simulink model "GFM_29bus"  (R2021a)
settings: Solver=ode1  StartTime=0.0  StopTime=4.5  FixedStep=Time_Step  RelTol=1e-3  EnableMultiTasking=on
PreLoadFcn:
  | Init_29bus;
InitFcn:
  | Init_29bus;
undefined symbols (not defined in the file): D1, D11, Delta, Time_Step, VSC01_Delta_P_Time_Step, VSC01_Delta_P_Value
libraries: spsSeriesRLCBranchLib x41, spsLoadFlowBusLib x28, spsDistributedParametersLineLib x19, spsThreePhaseSeriesRLCLoadLib x15, spsThreePhaseTransformerTwoWindingsLib x12, spsThreePhaseVIMeasurementLib x11, spsThreePhaseParallelRLCLoadLib x10, spsSynchronousMachinepuStandardLib x6, spsExcitationSystemLib x6, spsHydraulicTurbineandGovernorLib x6, spsGenericPowerSystemStabilizerLib x6, spsMultiBandPowerSystemStabilizerLib x6
(part 5 of 6)

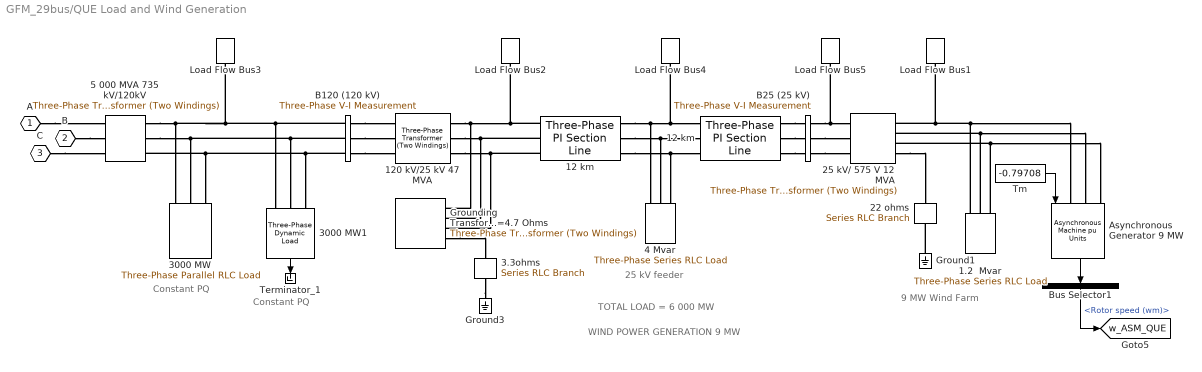
== system GFM_29bus/QUE Load and Wind Generation ==
  note: 9 MW Wind Farm
  note: 25 kV feeder
  note: Constant PQ
  note: Constant PQ
  note: WIND POWER GENERATION 9 MW
  note: TOTAL LOAD = 6 000 MW
  1.2  Mvar : spsThreePhaseSeriesRLCLoadLib/Three-Phase Series RLC Load  LConnTagsString=A|B|C  Configuration=Delta  NominalVoltage=575  Vabc=[1e3 1e3 1e3]  Vabcp=[1e3 1e3 1e3]  NominalFrequency=60  UnbalancedPower=off  ActivePower=1.2e6/50  InductivePower=0  CapacitivePower=1.2e6  Pabc=[10e3 9e3 11e3]  QLabc=[100 90 110]  QCabc=[100 90 110]  Pabcp=[10e3 9e3 11e3]  QLabcp=[100 90 110]  QCabcp=[100 90 110]  Measurements=None  LoadType=constant Z
  12 km : spsThreePhasePISectionLineLib/Three-Phase PI Section Line  LConnTagsString=a|b|c  RConnTagsString=A|B|C  Length=12  Frequency=60  Resistances=[0.1153 0.413]  Inductances=[1.05e-3 3.32e-3]  Capacitances=[11.33e-009 5.01e-009]
  "12 km " : spsThreePhasePISectionLineLib/Three-Phase PI Section Line  LConnTagsString=a|b|c  RConnTagsString=A|B|C  Length=12  Frequency=60  Resistances=[0.1153 0.413]  Inductances=[1.05e-3 3.32e-3]  Capacitances=[11.33e-009 5.01e-009]
  120 kV/25 kV 47 MVA : spsThreePhaseTransformerTwoWindingsLib/Three-Phase Transformer (Two Windings)  Winding1Connection=Yg  Winding2Connection=Delta (D1)  CoreType=Three single-phase transformers  SetSaturation=off  Hysteresis=off  DataFile='basic_model'  SetInitialFlux=off  Measurements=None  UNITS=pu  NominalPower=[47e6 60 ]  Winding1="[ 120e3  0.08/30   0.08 ]"  Winding2="[ 25e3  0.08/30  0.08]"  Rm=500  Lm=500  L0=0.5  Saturation="[ 0,0  ;  0.005,1.2  ;  1.0,1.4 ]"  InitialFluxes=[ 0.8 , -0.8 , 0.7 ]  BreakLoop=off  DiscreteSolver=Trapezoidal iterative  DataType=off  TransfoNumber=0
  "22 ohms " : spsSeriesRLCBranchLib/Series RLC Branch  LConnTagsString=__new0  RConnTagsString=__new0  BranchType=R  Resistance=22  Inductance=1.0  SetiL0=off  InitialCurrent=0  Capacitance=1.0  Setx0=off  InitialVoltage=0  Measurements=None
  25 kV/ 575 V 12 MVA : spsThreePhaseTransformerTwoWindingsLib/Three-Phase Transformer (Two Windings)  Winding1Connection=Yg  Winding2Connection=Yn  CoreType=Three single-phase transformers  SetSaturation=off  Hysteresis=off  DataFile='hysteresis'  SetInitialFlux=off  Measurements=None  UNITS=pu  NominalPower="[12e6  60]"  Winding1=[25e3 , 0.025/30 , 0.025]  Winding2=[ 575, 0.025/30 , 0.025]  Rm=500  Lm=inf  L0=0.5  Saturation=[ 0,0 ; 0.0024,1.2 ; 1.0,1.52 ]  InitialFluxes=[ 0.8 , -0.8 , 0.7 ]  BreakLoop=off  DiscreteSolver=Trapezoidal iterative  DataType=off  TransfoNumber=0
  "3.3ohms " : spsSeriesRLCBranchLib/Series RLC Branch  LConnTagsString=__new0  RConnTagsString=__new0  BranchType=R  Resistance=3.3  Inductance=1.0  SetiL0=off  InitialCurrent=0  Capacitance=1.0  Setx0=off  InitialVoltage=0  Measurements=None
  3000 MW : spsThreePhaseParallelRLCLoadLib/Three-Phase Parallel RLC Load  LConnTagsString=A|B|C  Configuration=Y (grounded)  NominalVoltage=(120000)*1.0062  Vabc=[1e3 1e3 1e3]  Vabcp=[1e3 1e3 1e3]  NominalFrequency=60  UnbalancedPower=off  ActivePower=3000000000  InductivePower=0  CapacitivePower=0  Pabc=[10e3 9e3 11e3]  QLabc=[100 90 110]  QCabc=[100 90 110]  Pabcp=[10e3 9e3 11e3]  QLabcp=[100 90 110]  QCabcp=[100 90 110]  Measurements=None  LoadType=constant PQ
  3000 MW1 : spsThreePhaseDynamicLoadLib/Three-Phase Dynamic Load  NominalVoltage=[ 120e3 60 ]  ActiveReactivePowers=[3e+09 0]  PositiveSequence=[1.0062 -46.9013]  ExternalControl=off  NpNq=[1.3 2]  TimeConstants="[0  0  0  0]"  MinimumVoltage=0.7  Tfilter=1e-4  LoadFlowParameters=[4,0,0,0,0]
      settings: SourceProductBaseCode=PS
  4 Mvar : spsThreePhaseSeriesRLCLoadLib/Three-Phase Series RLC Load  LConnTagsString=A|B|C  Configuration=Delta  NominalVoltage=25e3  Vabc=[1e3 1e3 1e3]  Vabcp=[1e3 1e3 1e3]  NominalFrequency=60  UnbalancedPower=off  ActivePower=0  InductivePower=0  CapacitivePower=4e6  Pabc=[10e3 9e3 11e3]  QLabc=[100 90 110]  QCabc=[100 90 110]  Pabcp=[10e3 9e3 11e3]  QLabcp=[100 90 110]  QCabcp=[100 90 110]  Measurements=None  LoadType=constant Z
  5 000 MVA 735 kV/120kV : spsThreePhaseTransformerTwoWindingsLib/Three-Phase Transformer (Two Windings)  Winding1Connection=Yg  Winding2Connection=Delta (D1)  CoreType=Three single-phase transformers  SetSaturation=off  Hysteresis=off  DataFile='basic_model'  SetInitialFlux=off  Measurements=None  UNITS=pu  NominalPower=[ 5000e6 60 ]  Winding1="[ 735e3 0.002  0.12]"  Winding2=[120e3 0.002 0]  Rm=500  Lm=500  L0=0.5  Saturation="[ 0,0  ;  0.005,1.2  ;  1.0,1.4 ]"  InitialFluxes=[ 0.8 , -0.8 , 0.7 ]  BreakLoop=off  DiscreteSolver=Trapezoidal iterative  DataType=off  TransfoNumber=0
  Asynchronous Generator 9 MW : spsAsynchronousMachinepuUnitsLib/Asynchronous Machine pu Units  RotorType=Squirrel-cage  PresetModel=No  MechanicalLoad=Torque Tm  ShowDetailedParameters=on  ReferenceFrame=Rotor  Units=pu  MeasurementBus=off  NominalParameters=[6*1.5e6/0.9 575 60]  VoltageRatio=1  Stator=[ 0.004843 0.1248]  Rotor=[ 0.004377 0.1791]  Cage1=[0.01909 0.0397]  Cage2=[0.01909 0.0397]  Lm=6.77  Mechanical="[5.04  0  3]"  PolePairs=3  InitialConditions=[-0.00366846 0 0.851241 0.851241 0.851241 136.952 16.9521 256.952]  SimulateSaturation=off  Saturation=[ 0 0 ; 0 0 ]  LoadFlowParameters=0  TsPowergui=0  TsBlock=-1  IterativeModel=Trapezoidal non iterative  IterativeDiscreteModel=Trapezoidal non iterative  Pmec=-8000000
      settings: SourceProductBaseCode=PS
  B120 (120 kV) : spsThreePhaseVIMeasurementLib/Three-Phase V-I Measurement  VoltageMeasurement=no  SetLabelV=on  LabelV=Vabc_B120  Vpu=on  VpuLL=off  CurrentMeasurement=no  SetLabelI=on  LabelI=Iabc_B120  Ipu=off  Pbase=100e6  Vbase=120e3  OutputType=Complex  PhasorSimulation=off  PSBequivalent=0
  B25 (25 kV) : spsThreePhaseVIMeasurementLib/Three-Phase V-I Measurement  VoltageMeasurement=no  SetLabelV=on  LabelV=Vabc_B25  Vpu=on  VpuLL=off  CurrentMeasurement=no  SetLabelI=on  LabelI=Iabc_B25  Ipu=on  Pbase=10e6  Vbase=25e3  OutputType=Complex  PhasorSimulation=off  PSBequivalent=0
  Bus Selector1 : BusSelector  OutputSignals=Mechanical.Rotor speed (wm)
  Ground1 : spsGroundLib/Ground  LConnTagsString=a
  Ground3 : spsGroundLib/Ground  LConnTagsString=a
  Grounding Transformer X0=4.7 Ohms : spsThreePhaseTransformerTwoWindingsLib/Three-Phase Transformer (Two Windings)  Winding1Connection=Yn  Winding2Connection=Delta (D11)  CoreType=Three single-phase transformers  SetSaturation=off  Hysteresis=off  DataFile='basic_model'  SetInitialFlux=off  Measurements=None  UNITS=pu  NominalPower=[100e6 60]  Winding1="[ 25e3  4.7/(25e3^2/100e6)/30    4.7/(25e3^2/100e6)]"  Winding2="[ 25e3  1e-6  0]"  Rm=500  Lm=500  L0=0.5  Saturation="[ 0,0  ;  0.005,1.2  ;  1.0,1.4 ]"  InitialFluxes=[ 0.8 , -0.8 , 0.7 ]  BreakLoop=off  DiscreteSolver=Trapezoidal iterative  DataType=off  TransfoNumber=0
  Load Flow Bus1 : spsLoadFlowBusLib/Load Flow Bus  LConnTagsString=a  Phases=single  Connectors=on one side  ID=QUE_575  Vbase=575  Vref=1  Vangle=0  VLF=1.021  VLFb=1  VLFc=1  angleLF=-67.07  angleLFb=0  angleLFc=0
      settings: AttributesFormatString=%<ID>\n%<Vbase>V\n%<VLF>pu\n%<angleLF>deg.  SourceProductBaseCode=PS
  Load Flow Bus2 : spsLoadFlowBusLib/Load Flow Bus  LConnTagsString=a  Phases=single  Connectors=on one side  ID=QUE_25_1  Vbase=25e3  Vref=1  Vangle=0  VLF=1.009  VLFb=1  VLFc=1  angleLF=-75.49  angleLFb=0  angleLFc=0
      settings: AttributesFormatString=%<ID>\n%<Vbase>V\n%<VLF>pu\n%<angleLF>deg.  SourceProductBaseCode=PS
  Load Flow Bus3 : spsLoadFlowBusLib/Load Flow Bus  LConnTagsString=a  Phases=single  Connectors=on one side  ID=QUE1  Vbase=120e3  Vref=1  Vangle=0  VLF=1.006  VLFb=1  VLFc=1  angleLF=-46.9  angleLFb=0  angleLFc=0
      settings: AttributesFormatString=%<ID>\n%<Vbase>V\n%<VLF>pu\n%<angleLF>deg.  SourceProductBaseCode=PS
  Load Flow Bus4 : spsLoadFlowBusLib/Load Flow Bus  LConnTagsString=a  Phases=single  Connectors=on one side  ID=QUE_25_2  Vbase=25e3  Vref=1  Vangle=0  VLF=1.033  VLFb=1  VLFc=1  angleLF=-72.41  angleLFb=0  angleLFc=0
      settings: AttributesFormatString=%<ID>\n%<Vbase>V\n%<VLF>pu\n%<angleLF>deg.  SourceProductBaseCode=PS
  Load Flow Bus5 : spsLoadFlowBusLib/Load Flow Bus  LConnTagsString=a  Phases=single  Connectors=on one side  ID=QUE_25_3  Vbase=25e3  Vref=1  Vangle=0  VLF=1.029  VLFb=1  VLFc=1  angleLF=-68.88  angleLFb=0  angleLFc=0
      settings: AttributesFormatString=%<ID>\n%<Vbase>V\n%<VLF>pu\n%<angleLF>deg.  SourceProductBaseCode=PS
  Terminator_1 : Terminator
  Tm : Constant  Value=-0.79708
  A : PMIOPort  Side=Left
  B : PMIOPort  Port=2  Side=Left
  C : PMIOPort  Port=3  Side=Left
  tag scope: w_ASM_QUE=global
  wires:
  Tm/1 -> Asynchronous Generator 9 MW/1
  Asynchronous Generator 9 MW/1 -> Bus Selector1/1
  Bus Selector1/1 -> [w_ASM_QUE]  "<Rotor speed (wm)>"
  3000 MW1/1 -> Terminator_1/1
  connections:
  B120 (120 kV)/RConn3 -- 120 kV/25 kV 47 MVA/LConn3
  B120 (120 kV)/RConn2 -- 120 kV/25 kV 47 MVA/LConn2
  B120 (120 kV)/RConn1 -- 120 kV/25 kV 47 MVA/LConn1
  A/RConn1 -- 5 000 MVA 735 kV/120kV/LConn1
  B/RConn1 -- 5 000 MVA 735 kV/120kV/LConn2
  C/RConn1 -- 5 000 MVA 735 kV/120kV/LConn3
  Load Flow Bus3/LConn1 -- B120 (120 kV)/LConn1 -- 3000 MW1/LConn1 -- 5 000 MVA 735 kV/120kV/RConn1 -- 3000 MW/LConn1
  B120 (120 kV)/LConn2 -- 5 000 MVA 735 kV/120kV/RConn2 -- 3000 MW/LConn2 -- 3000 MW1/LConn2
  B120 (120 kV)/LConn3 -- 5 000 MVA 735 kV/120kV/RConn3 -- 3000 MW/LConn3 -- 3000 MW1/LConn3
  12 km/LConn2 -- 120 kV/25 kV 47 MVA/RConn2 -- Grounding Transformer X0=4.7 Ohms/LConn2
  12 km/LConn3 -- 120 kV/25 kV 47 MVA/RConn3 -- Grounding Transformer X0=4.7 Ohms/LConn3
  Load Flow Bus2/LConn1 -- 12 km/LConn1 -- Grounding Transformer X0=4.7 Ohms/LConn1 -- 120 kV/25 kV 47 MVA/RConn1
  "3.3ohms "/RConn1 -- Ground3/LConn1
  Grounding Transformer X0=4.7 Ohms/LConn4 -- "3.3ohms "/LConn1
  25 kV/ 575 V 12 MVA/RConn4 -- "22 ohms "/LConn1
  Ground1/LConn1 -- "22 ohms "/RConn1
  Load Flow Bus1/LConn1 -- 1.2  Mvar/LConn1 -- Asynchronous Generator 9 MW/LConn1 -- 25 kV/ 575 V 12 MVA/RConn1
  1.2  Mvar/LConn2 -- 25 kV/ 575 V 12 MVA/RConn2 -- Asynchronous Generator 9 MW/LConn2
  1.2  Mvar/LConn3 -- 25 kV/ 575 V 12 MVA/RConn3 -- Asynchronous Generator 9 MW/LConn3
  B25 (25 kV)/RConn1 -- 25 kV/ 575 V 12 MVA/LConn1 -- Load Flow Bus5/LConn1
  B25 (25 kV)/RConn2 -- 25 kV/ 575 V 12 MVA/LConn2
  B25 (25 kV)/RConn3 -- 25 kV/ 575 V 12 MVA/LConn3
  "12 km "/RConn1 -- B25 (25 kV)/LConn1
  "12 km "/RConn2 -- B25 (25 kV)/LConn2
  "12 km "/RConn3 -- B25 (25 kV)/LConn3
  12 km/RConn1 -- "12 km "/LConn1 -- Load Flow Bus4/LConn1 -- 4 Mvar/LConn1
  12 km/RConn2 -- "12 km "/LConn2 -- 4 Mvar/LConn2
  12 km/RConn3 -- "12 km "/LConn3 -- 4 Mvar/LConn3

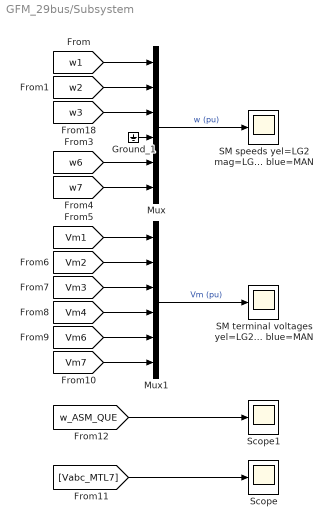
== system GFM_29bus/Subsystem ==
  Ground_1 : Ground
  Mux : Mux  Inputs=6
  Mux1 : Mux  Inputs=6
  "SM speeds yel=LG2 mag=LG3 cyan=LG4 red=MTL green=CHU blue=MAN " : Scope
  SM terminal voltages yel=LG2 mag=LG3 cyan=LG4 red=MTL green=CHU blue=MAN : Scope
  Scope : Scope
  Scope1 : Scope
  wires:
  [Vabc_MTL7] -> Scope/1
  [w_ASM_QUE] -> Scope1/1
  Mux/1 -> "SM speeds yel=LG2 mag=LG3 cyan=LG4 red=MTL green=CHU blue=MAN "/1  "w (pu)"
  [w1] -> Mux/1
  [w2] -> Mux/2
  [w7] -> Mux/6
  [w6] -> Mux/5
  [w3] -> Mux/3
  Mux1/1 -> SM terminal voltages yel=LG2 mag=LG3 cyan=LG4 red=MTL green=CHU blue=MAN/1  "Vm (pu)"
  [Vm1] -> Mux1/1
  [Vm2] -> Mux1/2
  [Vm7] -> Mux1/6
  [Vm6] -> Mux1/5
  [Vm4] -> Mux1/4
  [Vm3] -> Mux1/3
  Ground_1/1 -> Mux/4

== system GFM_29bus/Subsystem1 ==
  In1 : Inport
  Constant : Constant
  Sum : Sum  Inputs=|++  SaturateOnIntegerOverflow=on
  tag scope: PSS_select=global
  wires:
  In1/1 -> Sum/1
  Sum/1 -> [PSS_select]
  Constant/1 -> Sum/2

== system GFM_29bus/Subsystem2 ==

== system GFM_29bus/North-West Network/Cs  CHMN  ==
  note: B
  Ca : spsSeriesRLCBranchLib/Series RLC Branch  LConnTagsString=__new0  RConnTagsString=__new0  BranchType=C  Resistance=1.0  Inductance=1.0  SetiL0=off  InitialCurrent=0  Capacitance=Cs  Setx0=off  InitialVoltage=0  Measurements=None
  Cb : spsSeriesRLCBranchLib/Series RLC Branch  LConnTagsString=__new0  RConnTagsString=__new0  BranchType=C  Resistance=1.0  Inductance=1.0  SetiL0=off  InitialCurrent=0  Capacitance=Cs  Setx0=off  InitialVoltage=0  Measurements=None
  Cc : spsSeriesRLCBranchLib/Series RLC Branch  LConnTagsString=__new0  RConnTagsString=__new0  BranchType=C  Resistance=1.0  Inductance=1.0  SetiL0=off  InitialCurrent=0  Capacitance=Cs  Setx0=off  InitialVoltage=0  Measurements=None
  A : PMIOPort  Side=Left
  B : PMIOPort  Port=2  Side=Left
  C : PMIOPort  Port=3  Side=Left
  "A " : PMIOPort  Port=4  Side=Right
  "B " : PMIOPort  Port=5  Side=Right
  "C " : PMIOPort  Port=6  Side=Right
  connections:
  Cc/RConn1 -- "C "/RConn1
  C/RConn1 -- Cc/LConn1
  Cb/RConn1 -- "B "/RConn1
  B/RConn1 -- Cb/LConn1
  Ca/RConn1 -- "A "/RConn1
  A/RConn1 -- Ca/LConn1

== system GFM_29bus/North-West Network/Cs ABI+CHB  ==
  note: B
  Ca : spsSeriesRLCBranchLib/Series RLC Branch  LConnTagsString=__new0  RConnTagsString=__new0  BranchType=C  Resistance=1.0  Inductance=1.0  SetiL0=off  InitialCurrent=0  Capacitance=Cs  Setx0=off  InitialVoltage=0  Measurements=None
  Cb : spsSeriesRLCBranchLib/Series RLC Branch  LConnTagsString=__new0  RConnTagsString=__new0  BranchType=C  Resistance=1.0  Inductance=1.0  SetiL0=off  InitialCurrent=0  Capacitance=Cs  Setx0=off  InitialVoltage=0  Measurements=None
  Cc : spsSeriesRLCBranchLib/Series RLC Branch  LConnTagsString=__new0  RConnTagsString=__new0  BranchType=C  Resistance=1.0  Inductance=1.0  SetiL0=off  InitialCurrent=0  Capacitance=Cs  Setx0=off  InitialVoltage=0  Measurements=None
  A : PMIOPort  Side=Left
  B : PMIOPort  Port=2  Side=Left
  C : PMIOPort  Port=3  Side=Left
  "A " : PMIOPort  Port=4  Side=Right
  "B " : PMIOPort  Port=5  Side=Right
  "C " : PMIOPort  Port=6  Side=Right
  connections:
  Cc/RConn1 -- "C "/RConn1
  C/RConn1 -- Cc/LConn1
  Cb/RConn1 -- "B "/RConn1
  B/RConn1 -- Cb/LConn1
  Ca/RConn1 -- "A "/RConn1
  A/RConn1 -- Ca/LConn1

== system GFM_29bus/North-West Network/Cs ALB ==
  note: B
  Ca : spsSeriesRLCBranchLib/Series RLC Branch  LConnTagsString=__new0  RConnTagsString=__new0  BranchType=C  Resistance=1.0  Inductance=1.0  SetiL0=off  InitialCurrent=0  Capacitance=Cs  Setx0=off  InitialVoltage=0  Measurements=None
  Cb : spsSeriesRLCBranchLib/Series RLC Branch  LConnTagsString=__new0  RConnTagsString=__new0  BranchType=C  Resistance=1.0  Inductance=1.0  SetiL0=off  InitialCurrent=0  Capacitance=Cs  Setx0=off  InitialVoltage=0  Measurements=None
  Cc : spsSeriesRLCBranchLib/Series RLC Branch  LConnTagsString=__new0  RConnTagsString=__new0  BranchType=C  Resistance=1.0  Inductance=1.0  SetiL0=off  InitialCurrent=0  Capacitance=Cs  Setx0=off  InitialVoltage=0  Measurements=None
  A : PMIOPort  Side=Left
  B : PMIOPort  Port=2  Side=Left
  C : PMIOPort  Port=3  Side=Left
  "A " : PMIOPort  Port=4  Side=Right
  "B " : PMIOPort  Port=5  Side=Right
  "C " : PMIOPort  Port=6  Side=Right
  connections:
  A/RConn1 -- Ca/LConn1
  Ca/RConn1 -- "A "/RConn1
  B/RConn1 -- Cb/LConn1
  Cb/RConn1 -- "B "/RConn1
  C/RConn1 -- Cc/LConn1
  Cc/RConn1 -- "C "/RConn1

== system GFM_29bus/North-West Network/Cs LVDN  ==
  note: B
  Ca : spsSeriesRLCBranchLib/Series RLC Branch  LConnTagsString=__new0  RConnTagsString=__new0  BranchType=C  Resistance=1.0  Inductance=1.0  SetiL0=off  InitialCurrent=0  Capacitance=Cs  Setx0=off  InitialVoltage=0  Measurements=None
  Cb : spsSeriesRLCBranchLib/Series RLC Branch  LConnTagsString=__new0  RConnTagsString=__new0  BranchType=C  Resistance=1.0  Inductance=1.0  SetiL0=off  InitialCurrent=0  Capacitance=Cs  Setx0=off  InitialVoltage=0  Measurements=None
  Cc : spsSeriesRLCBranchLib/Series RLC Branch  LConnTagsString=__new0  RConnTagsString=__new0  BranchType=C  Resistance=1.0  Inductance=1.0  SetiL0=off  InitialCurrent=0  Capacitance=Cs  Setx0=off  InitialVoltage=0  Measurements=None
  A : PMIOPort  Side=Left
  B : PMIOPort  Port=2  Side=Left
  C : PMIOPort  Port=3  Side=Left
  "A " : PMIOPort  Port=4  Side=Right
  "B " : PMIOPort  Port=5  Side=Right
  "C " : PMIOPort  Port=6  Side=Right
  connections:
  A/RConn1 -- Ca/LConn1
  Ca/RConn1 -- "A "/RConn1
  B/RConn1 -- Cb/LConn1
  Cb/RConn1 -- "B "/RConn1
  C/RConn1 -- Cc/LConn1
  Cc/RConn1 -- "C "/RConn1

== system GFM_29bus/North-West Network/Cs LVDS  ==
  note: B
  Ca : spsSeriesRLCBranchLib/Series RLC Branch  LConnTagsString=__new0  RConnTagsString=__new0  BranchType=C  Resistance=1.0  Inductance=1.0  SetiL0=off  InitialCurrent=0  Capacitance=Cs  Setx0=off  InitialVoltage=0  Measurements=None
  Cb : spsSeriesRLCBranchLib/Series RLC Branch  LConnTagsString=__new0  RConnTagsString=__new0  BranchType=C  Resistance=1.0  Inductance=1.0  SetiL0=off  InitialCurrent=0  Capacitance=Cs  Setx0=off  InitialVoltage=0  Measurements=None
  Cc : spsSeriesRLCBranchLib/Series RLC Branch  LConnTagsString=__new0  RConnTagsString=__new0  BranchType=C  Resistance=1.0  Inductance=1.0  SetiL0=off  InitialCurrent=0  Capacitance=Cs  Setx0=off  InitialVoltage=0  Measurements=None
  A : PMIOPort  Side=Left
  B : PMIOPort  Port=2  Side=Left
  C : PMIOPort  Port=3  Side=Left
  "A " : PMIOPort  Port=4  Side=Right
  "B " : PMIOPort  Port=5  Side=Right
  "C " : PMIOPort  Port=6  Side=Right
  connections:
  Cc/RConn1 -- "C "/RConn1
  C/RConn1 -- Cc/LConn1
  Cb/RConn1 -- "B "/RConn1
  B/RConn1 -- Cb/LConn1
  Ca/RConn1 -- "A "/RConn1
  A/RConn1 -- Ca/LConn1

== system GFM_29bus/North-West Network/Cs NEM  ==
  note: B
  Ca : spsSeriesRLCBranchLib/Series RLC Branch  LConnTagsString=__new0  RConnTagsString=__new0  BranchType=C  Resistance=1.0  Inductance=1.0  SetiL0=off  InitialCurrent=0  Capacitance=Cs  Setx0=off  InitialVoltage=0  Measurements=None
  Cb : spsSeriesRLCBranchLib/Series RLC Branch  LConnTagsString=__new0  RConnTagsString=__new0  BranchType=C  Resistance=1.0  Inductance=1.0  SetiL0=off  InitialCurrent=0  Capacitance=Cs  Setx0=off  InitialVoltage=0  Measurements=None
  Cc : spsSeriesRLCBranchLib/Series RLC Branch  LConnTagsString=__new0  RConnTagsString=__new0  BranchType=C  Resistance=1.0  Inductance=1.0  SetiL0=off  InitialCurrent=0  Capacitance=Cs  Setx0=off  InitialVoltage=0  Measurements=None
  A : PMIOPort  Side=Left
  B : PMIOPort  Port=2  Side=Left
  C : PMIOPort  Port=3  Side=Left
  "A " : PMIOPort  Port=4  Side=Right
  "B " : PMIOPort  Port=5  Side=Right
  "C " : PMIOPort  Port=6  Side=Right
  connections:
  A/RConn1 -- Ca/LConn1
  Ca/RConn1 -- "A "/RConn1
  B/RConn1 -- Cb/LConn1
  Cb/RConn1 -- "B "/RConn1
  C/RConn1 -- Cc/LConn1
  Cc/RConn1 -- "C "/RConn1

== system GFM_29bus/North-West Network/Regulators1 ==
  m : Inport
  Bus Selector1 : BusSelector  OutputSignals="dq0 components.Stator voltage  vq (pu),dq0 components.Stator voltage  vd (pu),Mechanical.Rotor speed  wm  (pu),Output active power   Peo (pu)"
  Math Function1 : Math  Operator=hypot  SignedPower=on  SaturateOnIntegerOverflow=on
  Pref1 : Constant
  Turbine  & Excitation Regulators Mac2 : Subsystem
  Vref : Constant  Value=0.8201
  Pm : Outport  VectorParamsAs1DForOutWhenUnconnected=off
  Vf : Outport  Port=2  VectorParamsAs1DForOutWhenUnconnected=off
  tag scope: Vm1=global, w1=global
  wires:
  Pref1/1 -> Turbine  & Excitation Regulators Mac2/2(Vref)
  Turbine  & Excitation Regulators Mac2/1(Pm) -> Pm/1
  Vref/1 -> Turbine  & Excitation Regulators Mac2/1(Pref)
  Turbine  & Excitation Regulators Mac2/2(Vf) -> Vf/1
  Bus Selector1/1 -> Math Function1/1  "<Stator voltage  vq (pu)>"
  Bus Selector1/2 -> Math Function1/2  "<Stator voltage  vd (pu)>"
  Math Function1/1 -> Turbine  & Excitation Regulators Mac2/3(Vm), [Vm1]
  Bus Selector1/3 -> Turbine  & Excitation Regulators Mac2/4(w), [w1]  "<Rotor speed  wm  (pu)>"
  Bus Selector1/4 -> Turbine  & Excitation Regulators Mac2/5(Pe)  "<Output active power   Peo (pu)>"
  m/1 -> Bus Selector1/1

== system GFM_29bus/North-West Network/Regulators2 ==
  m : Inport
  Bus Selector1 : BusSelector  OutputSignals="dq0 components.Stator voltage  vq (pu),dq0 components.Stator voltage  vd (pu),Mechanical.Rotor speed  wm  (pu),Output active power   Peo (pu)"
  Math Function1 : Math  Operator=hypot  SignedPower=on  SaturateOnIntegerOverflow=on
  Pref1 : Constant
  Turbine  & Excitation Regulators Mac2 : Subsystem
  Vref : Constant  Value=0.81818
  Pm : Outport  VectorParamsAs1DForOutWhenUnconnected=off
  Vf : Outport  Port=2  VectorParamsAs1DForOutWhenUnconnected=off
  tag scope: Vm2=global, w2=global
  wires:
  m/1 -> Bus Selector1/1
  Bus Selector1/4 -> Turbine  & Excitation Regulators Mac2/5(Pe)  "<Output active power   Peo (pu)>"
  Bus Selector1/3 -> [w2], Turbine  & Excitation Regulators Mac2/4(w)  "<Rotor speed  wm  (pu)>"
  Math Function1/1 -> [Vm2], Turbine  & Excitation Regulators Mac2/3(Vm)
  Bus Selector1/2 -> Math Function1/2  "<Stator voltage  vd (pu)>"
  Bus Selector1/1 -> Math Function1/1  "<Stator voltage  vq (pu)>"
  Turbine  & Excitation Regulators Mac2/2(Vf) -> Vf/1
  Vref/1 -> Turbine  & Excitation Regulators Mac2/1(Pref)
  Turbine  & Excitation Regulators Mac2/1(Pm) -> Pm/1
  Pref1/1 -> Turbine  & Excitation Regulators Mac2/2(Vref)

== system GFM_29bus/North-West Network/Regulators3 ==
  m : Inport
  Bus Selector1 : BusSelector  OutputSignals="dq0 components.Stator voltage  vq (pu),dq0 components.Stator voltage  vd (pu),Mechanical.Rotor speed  wm  (pu),Output active power   Peo (pu)"
  Math Function1 : Math  Operator=hypot  SignedPower=on  SaturateOnIntegerOverflow=on
  Pref1 : Constant
  Turbine  & Excitation Regulators Mac2 : Subsystem
  Vref : Constant  Value=0.9
  Pm : Outport  VectorParamsAs1DForOutWhenUnconnected=off
  Vf : Outport  Port=2  VectorParamsAs1DForOutWhenUnconnected=off
  tag scope: Vm3=global, w3=global
  wires:
  Pref1/1 -> Turbine  & Excitation Regulators Mac2/2(Vref)
  Turbine  & Excitation Regulators Mac2/1(Pm) -> Pm/1
  Vref/1 -> Turbine  & Excitation Regulators Mac2/1(Pref)
  Turbine  & Excitation Regulators Mac2/2(Vf) -> Vf/1
  Bus Selector1/1 -> Math Function1/1  "<Stator voltage  vq (pu)>"
  Bus Selector1/2 -> Math Function1/2  "<Stator voltage  vd (pu)>"
  Math Function1/1 -> Turbine  & Excitation Regulators Mac2/3(Vm), [Vm3]
  Bus Selector1/3 -> Turbine  & Excitation Regulators Mac2/4(w), [w3]  "<Rotor speed  wm  (pu)>"
  Bus Selector1/4 -> Turbine  & Excitation Regulators Mac2/5(Pe)  "<Output active power   Peo (pu)>"
  m/1 -> Bus Selector1/1

== system GFM_29bus/North-West Network/Regulators4 ==
  m : Inport
  Bus Selector1 : BusSelector  OutputSignals="dq0 components.Stator voltage  vq (pu),dq0 components.Stator voltage  vd (pu),Mechanical.Rotor speed  wm  (pu),Output active power   Peo (pu)"
  Math Function1 : Math  Operator=hypot  SignedPower=on  SaturateOnIntegerOverflow=on
  Pref1 : Constant
  Turbine  & Excitation Regulators Mac2 : Subsystem
  Vref : Constant  Value=0.92593
  Pm : Outport  VectorParamsAs1DForOutWhenUnconnected=off
  Vf : Outport  Port=2  VectorParamsAs1DForOutWhenUnconnected=off
  tag scope: Vm4=global
  wires:
  m/1 -> Bus Selector1/1
  Bus Selector1/4 -> Turbine  & Excitation Regulators Mac2/5(Pe)  "<Output active power   Peo (pu)>"
  Bus Selector1/3 -> Turbine  & Excitation Regulators Mac2/4(w)  "<Rotor speed  wm  (pu)>"
  Math Function1/1 -> [Vm4], Turbine  & Excitation Regulators Mac2/3(Vm)
  Bus Selector1/2 -> Math Function1/2  "<Stator voltage  vd (pu)>"
  Bus Selector1/1 -> Math Function1/1  "<Stator voltage  vq (pu)>"
  Turbine  & Excitation Regulators Mac2/2(Vf) -> Vf/1
  Vref/1 -> Turbine  & Excitation Regulators Mac2/1(Pref)
  Turbine  & Excitation Regulators Mac2/1(Pm) -> Pm/1
  Pref1/1 -> Turbine  & Excitation Regulators Mac2/2(Vref)

== system GFM_29bus/North_East Network/Cs ARNS1  ==
  note: B
  Ca : spsSeriesRLCBranchLib/Series RLC Branch  LConnTagsString=__new0  RConnTagsString=__new0  BranchType=C  Resistance=1.0  Inductance=1.0  SetiL0=off  InitialCurrent=0  Capacitance=Cs  Setx0=off  InitialVoltage=0  Measurements=None
  Cb : spsSeriesRLCBranchLib/Series RLC Branch  LConnTagsString=__new0  RConnTagsString=__new0  BranchType=C  Resistance=1.0  Inductance=1.0  SetiL0=off  InitialCurrent=0  Capacitance=Cs  Setx0=off  InitialVoltage=0  Measurements=None
  Cc : spsSeriesRLCBranchLib/Series RLC Branch  LConnTagsString=__new0  RConnTagsString=__new0  BranchType=C  Resistance=1.0  Inductance=1.0  SetiL0=off  InitialCurrent=0  Capacitance=Cs  Setx0=off  InitialVoltage=0  Measurements=None
  A : PMIOPort  Side=Left
  B : PMIOPort  Port=2  Side=Left
  C : PMIOPort  Port=3  Side=Left
  "A " : PMIOPort  Port=4  Side=Right
  "B " : PMIOPort  Port=5  Side=Right
  "C " : PMIOPort  Port=6  Side=Right
  connections:
  Cc/RConn1 -- "C "/RConn1
  C/RConn1 -- Cc/LConn1
  Cb/RConn1 -- "B "/RConn1
  B/RConn1 -- Cb/LConn1
  Ca/RConn1 -- "A "/RConn1
  A/RConn1 -- Ca/LConn1

== system GFM_29bus/North_East Network/Cs ARNS2 ==
  note: B
  Ca : spsSeriesRLCBranchLib/Series RLC Branch  LConnTagsString=__new0  RConnTagsString=__new0  BranchType=C  Resistance=1.0  Inductance=1.0  SetiL0=off  InitialCurrent=0  Capacitance=Cs  Setx0=off  InitialVoltage=0  Measurements=None
  Cb : spsSeriesRLCBranchLib/Series RLC Branch  LConnTagsString=__new0  RConnTagsString=__new0  BranchType=C  Resistance=1.0  Inductance=1.0  SetiL0=off  InitialCurrent=0  Capacitance=Cs  Setx0=off  InitialVoltage=0  Measurements=None
  Cc : spsSeriesRLCBranchLib/Series RLC Branch  LConnTagsString=__new0  RConnTagsString=__new0  BranchType=C  Resistance=1.0  Inductance=1.0  SetiL0=off  InitialCurrent=0  Capacitance=Cs  Setx0=off  InitialVoltage=0  Measurements=None
  A : PMIOPort  Side=Left
  B : PMIOPort  Port=2  Side=Left
  C : PMIOPort  Port=3  Side=Left
  "A " : PMIOPort  Port=4  Side=Right
  "B " : PMIOPort  Port=5  Side=Right
  "C " : PMIOPort  Port=6  Side=Right
  connections:
  A/RConn1 -- Ca/LConn1
  Ca/RConn1 -- "A "/RConn1
  B/RConn1 -- Cb/LConn1
  Cb/RConn1 -- "B "/RConn1
  C/RConn1 -- Cc/LConn1
  Cc/RConn1 -- "C "/RConn1

== system GFM_29bus/North_East Network/Cs BER ==
  note: B
  Ca : spsSeriesRLCBranchLib/Series RLC Branch  LConnTagsString=__new0  RConnTagsString=__new0  BranchType=C  Resistance=1.0  Inductance=1.0  SetiL0=off  InitialCurrent=0  Capacitance=Cs  Setx0=off  InitialVoltage=0  Measurements=None
  Cb : spsSeriesRLCBranchLib/Series RLC Branch  LConnTagsString=__new0  RConnTagsString=__new0  BranchType=C  Resistance=1.0  Inductance=1.0  SetiL0=off  InitialCurrent=0  Capacitance=Cs  Setx0=off  InitialVoltage=0  Measurements=None
  Cc : spsSeriesRLCBranchLib/Series RLC Branch  LConnTagsString=__new0  RConnTagsString=__new0  BranchType=C  Resistance=1.0  Inductance=1.0  SetiL0=off  InitialCurrent=0  Capacitance=Cs  Setx0=off  InitialVoltage=0  Measurements=None
  A : PMIOPort  Side=Left
  B : PMIOPort  Port=2  Side=Left
  C : PMIOPort  Port=3  Side=Left
  "A " : PMIOPort  Port=4  Side=Right
  "B " : PMIOPort  Port=5  Side=Right
  "C " : PMIOPort  Port=6  Side=Right
  connections:
  Cc/RConn1 -- "C "/RConn1
  C/RConn1 -- Cc/LConn1
  Cb/RConn1 -- "B "/RConn1
  B/RConn1 -- Cb/LConn1
  Ca/RConn1 -- "A "/RConn1
  A/RConn1 -- Ca/LConn1

== system GFM_29bus/North_East Network/Cs MTG+ARNN  ==
  note: B
  Ca : spsSeriesRLCBranchLib/Series RLC Branch  LConnTagsString=__new0  RConnTagsString=__new0  BranchType=C  Resistance=1.0  Inductance=1.0  SetiL0=off  InitialCurrent=0  Capacitance=Cs  Setx0=off  InitialVoltage=0  Measurements=None
  Cb : spsSeriesRLCBranchLib/Series RLC Branch  LConnTagsString=__new0  RConnTagsString=__new0  BranchType=C  Resistance=1.0  Inductance=1.0  SetiL0=off  InitialCurrent=0  Capacitance=Cs  Setx0=off  InitialVoltage=0  Measurements=None
  Cc : spsSeriesRLCBranchLib/Series RLC Branch  LConnTagsString=__new0  RConnTagsString=__new0  BranchType=C  Resistance=1.0  Inductance=1.0  SetiL0=off  InitialCurrent=0  Capacitance=Cs  Setx0=off  InitialVoltage=0  Measurements=None
  A : PMIOPort  Side=Left
  B : PMIOPort  Port=2  Side=Left
  C : PMIOPort  Port=3  Side=Left
  "A " : PMIOPort  Port=4  Side=Right
  "B " : PMIOPort  Port=5  Side=Right
  "C " : PMIOPort  Port=6  Side=Right
  connections:
  A/RConn1 -- Ca/LConn1
  Ca/RConn1 -- "A "/RConn1
  B/RConn1 -- Cb/LConn1
  Cb/RConn1 -- "B "/RConn1
  C/RConn1 -- Cc/LConn1
  Cc/RConn1 -- "C "/RConn1

== system GFM_29bus/North_East Network/Cs PER  ==
  note: B
  Ca : spsSeriesRLCBranchLib/Series RLC Branch  LConnTagsString=__new0  RConnTagsString=__new0  BranchType=C  Resistance=1.0  Inductance=1.0  SetiL0=off  InitialCurrent=0  Capacitance=Cs  Setx0=off  InitialVoltage=0  Measurements=None
  Cb : spsSeriesRLCBranchLib/Series RLC Branch  LConnTagsString=__new0  RConnTagsString=__new0  BranchType=C  Resistance=1.0  Inductance=1.0  SetiL0=off  InitialCurrent=0  Capacitance=Cs  Setx0=off  InitialVoltage=0  Measurements=None
  Cc : spsSeriesRLCBranchLib/Series RLC Branch  LConnTagsString=__new0  RConnTagsString=__new0  BranchType=C  Resistance=1.0  Inductance=1.0  SetiL0=off  InitialCurrent=0  Capacitance=Cs  Setx0=off  InitialVoltage=0  Measurements=None
  A : PMIOPort  Side=Left
  B : PMIOPort  Port=2  Side=Left
  C : PMIOPort  Port=3  Side=Left
  "A " : PMIOPort  Port=4  Side=Right
  "B " : PMIOPort  Port=5  Side=Right
  "C " : PMIOPort  Port=6  Side=Right
  connections:
  A/RConn1 -- Ca/LConn1
  Ca/RConn1 -- "A "/RConn1
  B/RConn1 -- Cb/LConn1
  Cb/RConn1 -- "B "/RConn1
  C/RConn1 -- Cc/LConn1
  Cc/RConn1 -- "C "/RConn1

== system GFM_29bus/North_East Network/Regulateurs6 ==
  m : Inport
  Bus Selector1 : BusSelector  OutputSignals="dq0 components.Stator voltage  vq (pu),dq0 components.Stator voltage  vd (pu),Mechanical.Rotor speed  wm  (pu),Output active power   Peo (pu)"
  Math Function1 : Math  Operator=hypot  SignedPower=on  SaturateOnIntegerOverflow=on
  Pref1 : Constant
  Turbine  & Excitation Regulators Mac2 : Subsystem
  Vref : Constant  Value=0.89286
  Pm : Outport  VectorParamsAs1DForOutWhenUnconnected=off
  Vf : Outport  Port=2  VectorParamsAs1DForOutWhenUnconnected=off
  tag scope: Vm6=global, w6=global
  wires:
  Pref1/1 -> Turbine  & Excitation Regulators Mac2/2(Vref)
  Turbine  & Excitation Regulators Mac2/1(Pm) -> Pm/1
  Vref/1 -> Turbine  & Excitation Regulators Mac2/1(Pref)
  Turbine  & Excitation Regulators Mac2/2(Vf) -> Vf/1
  Bus Selector1/1 -> Math Function1/1  "<Stator voltage  vq (pu)>"
  Bus Selector1/2 -> Math Function1/2  "<Stator voltage  vd (pu)>"
  Math Function1/1 -> Turbine  & Excitation Regulators Mac2/3(Vm), [Vm6]
  Bus Selector1/3 -> Turbine  & Excitation Regulators Mac2/4(w), [w6]  "<Rotor speed  wm  (pu)>"
  Bus Selector1/4 -> Turbine  & Excitation Regulators Mac2/5(Pe)  "<Output active power   Peo (pu)>"
  m/1 -> Bus Selector1/1

== system GFM_29bus/North_East Network/Regulateurs7 ==
  m : Inport
  Bus Selector1 : BusSelector  OutputSignals="dq0 components.Stator voltage  vq (pu),dq0 components.Stator voltage  vd (pu),Mechanical.Rotor speed  wm  (pu),Output active power   Peo (pu)"
  Math Function1 : Math  Operator=hypot  SignedPower=on  SaturateOnIntegerOverflow=on
  Pref1 : Constant
  Turbine  & Excitation Regulators Mac2 : Subsystem
  Vref : Constant  Value=0.9
  Pm : Outport  VectorParamsAs1DForOutWhenUnconnected=off
  Vf : Outport  Port=2  VectorParamsAs1DForOutWhenUnconnected=off
  tag scope: Vm7=global, w7=global
  wires:
  m/1 -> Bus Selector1/1
  Bus Selector1/4 -> Turbine  & Excitation Regulators Mac2/5(Pe)  "<Output active power   Peo (pu)>"
  Bus Selector1/3 -> Turbine  & Excitation Regulators Mac2/4(w), [w7]  "<Rotor speed  wm  (pu)>"
  Math Function1/1 -> [Vm7], Turbine  & Excitation Regulators Mac2/3(Vm)
  Bus Selector1/2 -> Math Function1/2  "<Stator voltage  vd (pu)>"
  Bus Selector1/1 -> Math Function1/1  "<Stator voltage  vq (pu)>"
  Turbine  & Excitation Regulators Mac2/2(Vf) -> Vf/1
  Vref/1 -> Turbine  & Excitation Regulators Mac2/1(Pref)
  Turbine  & Excitation Regulators Mac2/1(Pm) -> Pm/1
  Pref1/1 -> Turbine  & Excitation Regulators Mac2/2(Vref)

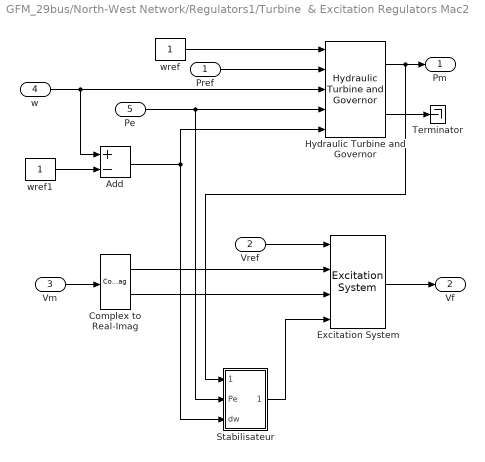
== system GFM_29bus/North-West Network/Regulators1/Turbine  & Excitation Regulators Mac2 ==
  Pref : Inport
  Vref : Inport  Port=2
  Vm : Inport  Port=3
  w : Inport  Port=4
  Pe : Inport  Port=5
  Add : Sum  Inputs=+-
  Complex to Real-Imag : ComplexToRealImag
  Excitation System : spsExcitationSystemLib/Excitation System  tr=20e-3  reg=[ 300, 0.001 ]  exc=[ 1, 0 ]  tgr=[ 0, 0 ]  damp=[ 0.001, 0.1 ]  sat=[ 0, 0 ]  lim=[ -11.5, 11.5, 0 ]  v0=[1 1.2551]
      settings: SourceProductBaseCode=PS
  Hydraulic Turbine and Governor : spsHydraulicTurbineandGovernorLib/Hydraulic Turbine and Governor  sm="[ 10/3  0.07 ]"  gate="[  0.01  0.97518  -0.1  0.1 ]"  reg="[  0.05 1.163  0.105  0  0.01  ]"  hyd="[  0  2.67  ]"  dref=0  po=0.82203
      settings: SourceProductBaseCode=PS
  Stabilisateur : Subsystem
  Terminator : Terminator
  wref : Constant
  wref1 : Constant
  Pm : Outport  VectorParamsAs1DForOutWhenUnconnected=off
  Vf : Outport  Port=2  VectorParamsAs1DForOutWhenUnconnected=off
  wires:
  Hydraulic Turbine and Governor/2 -> Terminator/1
  Hydraulic Turbine and Governor/1 -> Pm/1, Stabilisateur/1(Pm)
  Excitation System/1 -> Vf/1
  Pe/1 -> Hydraulic Turbine and Governor/4, Stabilisateur/2(Pe)
  Pref/1 -> Hydraulic Turbine and Governor/2
  Vref/1 -> Excitation System/1
  wref/1 -> Hydraulic Turbine and Governor/1
  w/1 -> Hydraulic Turbine and Governor/3, Add/1
  Vm/1 -> Complex to Real-Imag/1
  Complex to Real-Imag/2 -> Excitation System/3
  Complex to Real-Imag/1 -> Excitation System/2
  wref1/1 -> Add/2
  Add/1 -> Hydraulic Turbine and Governor/5, Stabilisateur/3(dw)
  Stabilisateur/1(Stab) -> Excitation System/4

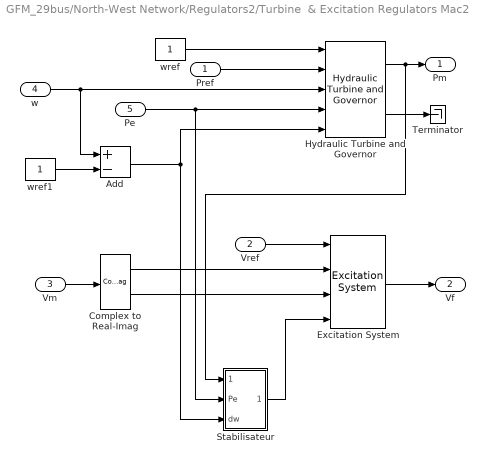
== system GFM_29bus/North-West Network/Regulators2/Turbine  & Excitation Regulators Mac2 ==
  Pref : Inport
  Vref : Inport  Port=2
  Vm : Inport  Port=3
  w : Inport  Port=4
  Pe : Inport  Port=5
  Add : Sum  Inputs=+-
  Complex to Real-Imag : ComplexToRealImag
  Excitation System : spsExcitationSystemLib/Excitation System  tr=20e-3  reg=[ 300, 0.001 ]  exc=[ 1, 0 ]  tgr=[ 0, 0 ]  damp=[ 0.001, 0.1 ]  sat=[ 0, 0 ]  lim=[ -11.5, 11.5, 0 ]  v0=[1 1.3376]
      settings: SourceProductBaseCode=PS
  Hydraulic Turbine and Governor : spsHydraulicTurbineandGovernorLib/Hydraulic Turbine and Governor  sm="[ 10/3  0.07 ]"  gate="[  0.01  0.97518  -0.1  0.1 ]"  reg="[  0.05 1.163  0.105  0  0.01  ]"  hyd="[  0  2.67  ]"  dref=0  po=0.82009
      settings: SourceProductBaseCode=PS
  Stabilisateur : Subsystem
  Terminator : Terminator
  wref : Constant
  wref1 : Constant
  Pm : Outport  VectorParamsAs1DForOutWhenUnconnected=off
  Vf : Outport  Port=2  VectorParamsAs1DForOutWhenUnconnected=off
  wires:
  Stabilisateur/1(Stab) -> Excitation System/4
  Add/1 -> Stabilisateur/3(dw), Hydraulic Turbine and Governor/5
  wref1/1 -> Add/2
  Complex to Real-Imag/1 -> Excitation System/2
  Complex to Real-Imag/2 -> Excitation System/3
  Vm/1 -> Complex to Real-Imag/1
  w/1 -> Add/1, Hydraulic Turbine and Governor/3
  wref/1 -> Hydraulic Turbine and Governor/1
  Vref/1 -> Excitation System/1
  Pref/1 -> Hydraulic Turbine and Governor/2
  Pe/1 -> Stabilisateur/2(Pe), Hydraulic Turbine and Governor/4
  Excitation System/1 -> Vf/1
  Hydraulic Turbine and Governor/1 -> Stabilisateur/1(Pm), Pm/1
  Hydraulic Turbine and Governor/2 -> Terminator/1

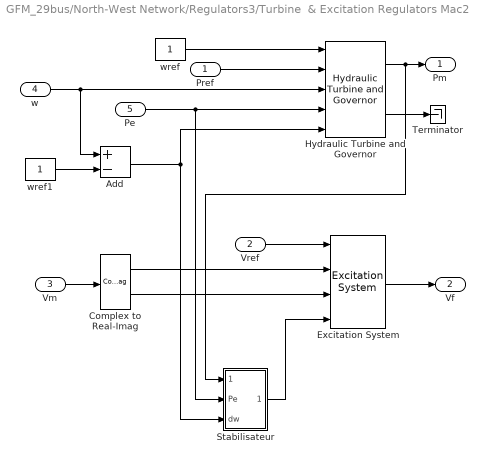
== system GFM_29bus/North-West Network/Regulators3/Turbine  & Excitation Regulators Mac2 ==
  Pref : Inport
  Vref : Inport  Port=2
  Vm : Inport  Port=3
  w : Inport  Port=4
  Pe : Inport  Port=5
  Add : Sum  Inputs=+-
  Complex to Real-Imag : ComplexToRealImag
  Excitation System : spsExcitationSystemLib/Excitation System  tr=20e-3  reg=[ 300, 0.001 ]  exc=[ 1, 0 ]  tgr=[ 0, 0 ]  damp=[ 0.001, 0.1 ]  sat=[ 0, 0 ]  lim=[ -11.5, 11.5, 0 ]  v0=[1 1.4051]
      settings: SourceProductBaseCode=PS
  Hydraulic Turbine and Governor : spsHydraulicTurbineandGovernorLib/Hydraulic Turbine and Governor  sm="[ 10/3  0.07 ]"  gate="[  0.01  0.97518  -0.1  0.1 ]"  reg="[  0.05 1.163  0.105  0  0.01  ]"  hyd="[  0  2.67  ]"  dref=0  po=0.90231
      settings: SourceProductBaseCode=PS
  Stabilisateur : Subsystem
  Terminator : Terminator
  wref : Constant
  wref1 : Constant
  Pm : Outport  VectorParamsAs1DForOutWhenUnconnected=off
  Vf : Outport  Port=2  VectorParamsAs1DForOutWhenUnconnected=off
  wires:
  Hydraulic Turbine and Governor/2 -> Terminator/1
  Hydraulic Turbine and Governor/1 -> Pm/1, Stabilisateur/1(Pm)
  Excitation System/1 -> Vf/1
  Pe/1 -> Hydraulic Turbine and Governor/4, Stabilisateur/2(Pe)
  Pref/1 -> Hydraulic Turbine and Governor/2
  Vref/1 -> Excitation System/1
  wref/1 -> Hydraulic Turbine and Governor/1
  w/1 -> Hydraulic Turbine and Governor/3, Add/1
  Vm/1 -> Complex to Real-Imag/1
  Complex to Real-Imag/2 -> Excitation System/3
  Complex to Real-Imag/1 -> Excitation System/2
  wref1/1 -> Add/2
  Add/1 -> Hydraulic Turbine and Governor/5, Stabilisateur/3(dw)
  Stabilisateur/1(Stab) -> Excitation System/4

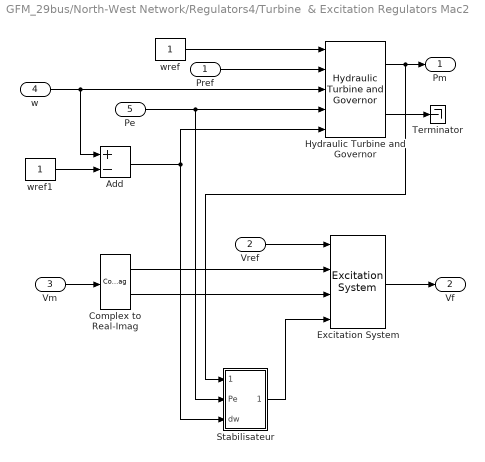
== system GFM_29bus/North-West Network/Regulators4/Turbine  & Excitation Regulators Mac2 ==
  Pref : Inport
  Vref : Inport  Port=2
  Vm : Inport  Port=3
  w : Inport  Port=4
  Pe : Inport  Port=5
  Add : Sum  Inputs=+-
  Complex to Real-Imag : ComplexToRealImag
  Excitation System : spsExcitationSystemLib/Excitation System  tr=20e-3  reg=[ 300, 0.001 ]  exc=[ 1, 0 ]  tgr=[ 0, 0 ]  damp=[ 0.001, 0.1 ]  sat=[ 0, 0 ]  lim=[ -11.5, 11.5, 0 ]  v0=[1 1.3322]
      settings: SourceProductBaseCode=PS
  Hydraulic Turbine and Governor : spsHydraulicTurbineandGovernorLib/Hydraulic Turbine and Governor  sm="[ 10/3  0.07 ]"  gate="[  0.01  0.97518  -0.1  0.1 ]"  reg="[  0.05 1.163  0.105  0  0.01  ]"  hyd="[  0  2.67  ]"  dref=0  po=0.92839
      settings: SourceProductBaseCode=PS
  Stabilisateur : Subsystem
  Terminator : Terminator
  wref : Constant
  wref1 : Constant
  Pm : Outport  VectorParamsAs1DForOutWhenUnconnected=off
  Vf : Outport  Port=2  VectorParamsAs1DForOutWhenUnconnected=off
  wires:
  Stabilisateur/1(Stab) -> Excitation System/4
  Add/1 -> Stabilisateur/3(dw), Hydraulic Turbine and Governor/5
  wref1/1 -> Add/2
  Complex to Real-Imag/1 -> Excitation System/2
  Complex to Real-Imag/2 -> Excitation System/3
  Vm/1 -> Complex to Real-Imag/1
  w/1 -> Add/1, Hydraulic Turbine and Governor/3
  wref/1 -> Hydraulic Turbine and Governor/1
  Vref/1 -> Excitation System/1
  Pref/1 -> Hydraulic Turbine and Governor/2
  Pe/1 -> Stabilisateur/2(Pe), Hydraulic Turbine and Governor/4
  Excitation System/1 -> Vf/1
  Hydraulic Turbine and Governor/1 -> Stabilisateur/1(Pm), Pm/1
  Hydraulic Turbine and Governor/2 -> Terminator/1

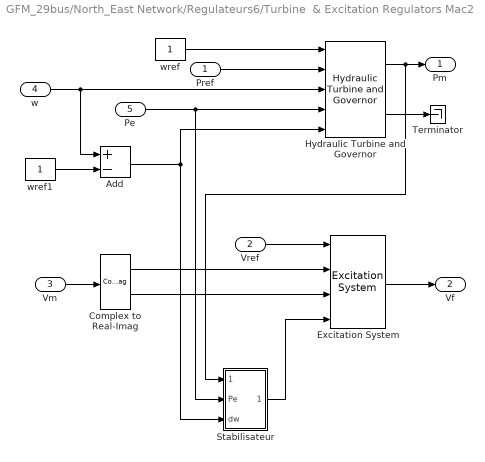
== system GFM_29bus/North_East Network/Regulateurs6/Turbine  & Excitation Regulators Mac2 ==
  Pref : Inport
  Vref : Inport  Port=2
  Vm : Inport  Port=3
  w : Inport  Port=4
  Pe : Inport  Port=5
  Add : Sum  Inputs=+-
  Complex to Real-Imag : ComplexToRealImag
  Excitation System : spsExcitationSystemLib/Excitation System  tr=20e-3  reg=[ 300, 0.001 ]  exc=[ 1, 0 ]  tgr=[ 0, 0 ]  damp=[ 0.001, 0.1 ]  sat=[ 0, 0 ]  lim=[ -11.5, 11.5, 0 ]  v0=[1 1.313]
      settings: SourceProductBaseCode=PS
  Hydraulic Turbine and Governor : spsHydraulicTurbineandGovernorLib/Hydraulic Turbine and Governor  sm="[ 10/3  0.07 ]"  gate="[  0.01  0.97518  -0.1  0.1 ]"  reg="[  0.05 1.163  0.105  0  0.01  ]"  hyd="[  0  2.67  ]"  dref=0  po=0.89514
      settings: SourceProductBaseCode=PS
  Stabilisateur : Subsystem
  Terminator : Terminator
  wref : Constant
  wref1 : Constant
  Pm : Outport  VectorParamsAs1DForOutWhenUnconnected=off
  Vf : Outport  Port=2  VectorParamsAs1DForOutWhenUnconnected=off
  wires:
  Hydraulic Turbine and Governor/2 -> Terminator/1
  Hydraulic Turbine and Governor/1 -> Pm/1, Stabilisateur/1(Pm)
  Excitation System/1 -> Vf/1
  Pe/1 -> Hydraulic Turbine and Governor/4, Stabilisateur/2(Pe)
  Pref/1 -> Hydraulic Turbine and Governor/2
  Vref/1 -> Excitation System/1
  wref/1 -> Hydraulic Turbine and Governor/1
  w/1 -> Hydraulic Turbine and Governor/3, Add/1
  Vm/1 -> Complex to Real-Imag/1
  Complex to Real-Imag/2 -> Excitation System/3
  Complex to Real-Imag/1 -> Excitation System/2
  wref1/1 -> Add/2
  Add/1 -> Hydraulic Turbine and Governor/5, Stabilisateur/3(dw)
  Stabilisateur/1(Stab) -> Excitation System/4

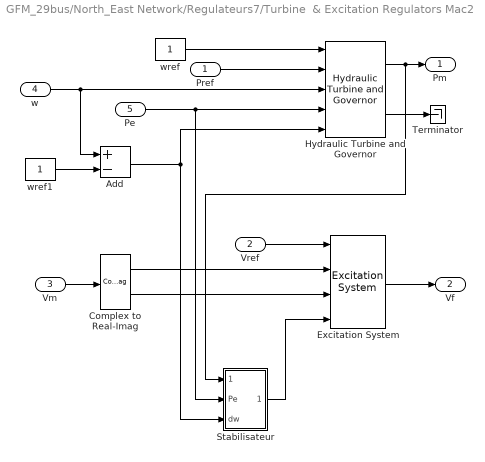
== system GFM_29bus/North_East Network/Regulateurs7/Turbine  & Excitation Regulators Mac2 ==
  Pref : Inport
  Vref : Inport  Port=2
  Vm : Inport  Port=3
  w : Inport  Port=4
  Pe : Inport  Port=5
  Add : Sum  Inputs=+-
  Complex to Real-Imag : ComplexToRealImag
  Excitation System : spsExcitationSystemLib/Excitation System  tr=20e-3  reg=[ 300, 0.001 ]  exc=[ 1, 0 ]  tgr=[ 0, 0 ]  damp=[ 0.001, 0.1 ]  sat=[ 0, 0 ]  lim=[ -11.5, 11.5, 0 ]  v0=[1 1.2555]
      settings: SourceProductBaseCode=PS
  Hydraulic Turbine and Governor : spsHydraulicTurbineandGovernorLib/Hydraulic Turbine and Governor  sm="[ 10/3  0.07 ]"  gate="[  0.01  0.97518  -0.1  0.1 ]"  reg="[  0.05 1.163  0.105  0  0.01  ]"  hyd="[  0  2.67  ]"  dref=0  po=0.90235
      settings: SourceProductBaseCode=PS
  Stabilisateur : Subsystem
  Terminator : Terminator
  wref : Constant
  wref1 : Constant
  Pm : Outport  VectorParamsAs1DForOutWhenUnconnected=off
  Vf : Outport  Port=2  VectorParamsAs1DForOutWhenUnconnected=off
  wires:
  Stabilisateur/1(Stab) -> Excitation System/4
  Add/1 -> Stabilisateur/3(dw), Hydraulic Turbine and Governor/5
  wref1/1 -> Add/2
  Complex to Real-Imag/1 -> Excitation System/2
  Complex to Real-Imag/2 -> Excitation System/3
  Vm/1 -> Complex to Real-Imag/1
  w/1 -> Add/1, Hydraulic Turbine and Governor/3
  wref/1 -> Hydraulic Turbine and Governor/1
  Vref/1 -> Excitation System/1
  Pref/1 -> Hydraulic Turbine and Governor/2
  Pe/1 -> Stabilisateur/2(Pe), Hydraulic Turbine and Governor/4
  Excitation System/1 -> Vf/1
  Hydraulic Turbine and Governor/1 -> Stabilisateur/1(Pm), Pm/1
  Hydraulic Turbine and Governor/2 -> Terminator/1

== system GFM_29bus/North-West Network/Regulators1/Turbine  & Excitation Regulators Mac2/Stabilisateur ==
  Pm : Inport
  Pe : Inport  Port=2
  dw : Inport  Port=3
  Generic Power System Stabilizer : spsGenericPowerSystemStabilizerLib/Generic Power System Stabilizer  Tsensor=15e-3  K=2.5  Twashout=1  Tleadlag1="[0.06  1]"  Tleadlag2="[0  0]"  VSlimits=[-0.15 0.15]  Vinit=0  Plot_On=off  MagdB_On=on  FreqRange=logspace(-2,2,500)
      settings: SourceProductBaseCode=PS
  Ground1 : Ground
  Multi-Band Power System Stabilizer : spsMultiBandPowerSystemStabilizerLib/Multi-Band Power System Stabilizer  OperationMode=Simplified settings  Kg=0.7  GL=[0.2 10]  GI=[0.9 30]  GH=[12.0 115]  GLd=[66 66 9.4]  TcLF=[1.667 2 0 0 0 0 2 2.4 0 0 0 0 1 1]  GId=[66 66 47.6]  TcIF=[1 1 0.25 0.3 0 0 1 1 0.3 0.36 0 0 0 0]  GHd=[66 66 233]  TcHF="[0.01 0.012 0 0 0 0  0.012 0.0144 0 0 0 0 1 1]"  LIM=[.075 .15 .15 .15]  Plot_On=off  MagdB_On=on  FreqRange=logspace(-2,2,500)
      settings: SourceProductBaseCode=PS
  Multiport Switch : MultiPortSwitch  SaturateOnIntegerOverflow=on  InputSameDT=on
  Sum2 : Sum  Inputs=+-  InputSameDT=on  SaturateOnIntegerOverflow=on  OutDataTypeStr=Inherit: Same as first input
  Stab : Outport  InitialOutput=0  VectorParamsAs1DForOutWhenUnconnected=off
  wires:
  Multiport Switch/1 -> Stab/1
  Generic Power System Stabilizer/1 -> Multiport Switch/3
  Sum2/1 -> Generic Power System Stabilizer/1
  Pm/1 -> Sum2/1
  Pe/1 -> Sum2/2
  Ground1/1 -> Multiport Switch/2
  [PSS_select] -> Multiport Switch/1
  dw/1 -> Multi-Band Power System Stabilizer/1
  Multi-Band Power System Stabilizer/1 -> Multiport Switch/4

== system GFM_29bus/North-West Network/Regulators2/Turbine  & Excitation Regulators Mac2/Stabilisateur ==
  Pm : Inport
  Pe : Inport  Port=2
  dw : Inport  Port=3
  Generic Power System Stabilizer : spsGenericPowerSystemStabilizerLib/Generic Power System Stabilizer  Tsensor=15e-3  K=2.5  Twashout=1  Tleadlag1="[0.06  1]"  Tleadlag2="[0  0]"  VSlimits=[-0.15 0.15]  Vinit=0  Plot_On=off  MagdB_On=on  FreqRange=logspace(-2,2,500)
      settings: SourceProductBaseCode=PS
  Ground1 : Ground
  Multi-Band Power System Stabilizer : spsMultiBandPowerSystemStabilizerLib/Multi-Band Power System Stabilizer  OperationMode=Simplified settings  Kg=0.7  GL=[0.2 10]  GI=[0.9 30]  GH=[12.0 115]  GLd=[66 66 9.4]  TcLF=[1.667 2 0 0 0 0 2 2.4 0 0 0 0 1 1]  GId=[66 66 47.6]  TcIF=[1 1 0.25 0.3 0 0 1 1 0.3 0.36 0 0 0 0]  GHd=[66 66 233]  TcHF="[0.01 0.012 0 0 0 0  0.012 0.0144 0 0 0 0 1 1]"  LIM=[.075 .15 .15 .15]  Plot_On=off  MagdB_On=on  FreqRange=logspace(-2,2,500)
      settings: SourceProductBaseCode=PS
  Multiport Switch : MultiPortSwitch  SaturateOnIntegerOverflow=on  InputSameDT=on
  Sum2 : Sum  Inputs=+-  InputSameDT=on  SaturateOnIntegerOverflow=on  OutDataTypeStr=Inherit: Same as first input
  Stab : Outport  InitialOutput=0  VectorParamsAs1DForOutWhenUnconnected=off
  wires:
  dw/1 -> Multi-Band Power System Stabilizer/1
  [PSS_select] -> Multiport Switch/1
  Ground1/1 -> Multiport Switch/2
  Pe/1 -> Sum2/2
  Pm/1 -> Sum2/1
  Sum2/1 -> Generic Power System Stabilizer/1
  Generic Power System Stabilizer/1 -> Multiport Switch/3
  Multiport Switch/1 -> Stab/1
  Multi-Band Power System Stabilizer/1 -> Multiport Switch/4

== system GFM_29bus/North-West Network/Regulators3/Turbine  & Excitation Regulators Mac2/Stabilisateur ==
  Pm : Inport
  Pe : Inport  Port=2
  dw : Inport  Port=3
  Generic Power System Stabilizer : spsGenericPowerSystemStabilizerLib/Generic Power System Stabilizer  Tsensor=15e-3  K=2.5  Twashout=1  Tleadlag1="[0.06  1]"  Tleadlag2="[0  0]"  VSlimits=[-0.15 0.15]  Vinit=0  Plot_On=off  MagdB_On=on  FreqRange=logspace(-2,2,500)
      settings: SourceProductBaseCode=PS
  Ground1 : Ground
  Multi-Band Power System Stabilizer : spsMultiBandPowerSystemStabilizerLib/Multi-Band Power System Stabilizer  OperationMode=Simplified settings  Kg=0.7  GL=[0.2 10]  GI=[0.9 30]  GH=[12.0 115]  GLd=[66 66 9.4]  TcLF=[1.667 2 0 0 0 0 2 2.4 0 0 0 0 1 1]  GId=[66 66 47.6]  TcIF=[1 1 0.25 0.3 0 0 1 1 0.3 0.36 0 0 0 0]  GHd=[66 66 233]  TcHF="[0.01 0.012 0 0 0 0  0.012 0.0144 0 0 0 0 1 1]"  LIM=[.075 .15 .15 .15]  Plot_On=off  MagdB_On=on  FreqRange=logspace(-2,2,500)
      settings: SourceProductBaseCode=PS
  Multiport Switch : MultiPortSwitch  SaturateOnIntegerOverflow=on  InputSameDT=on
  Sum2 : Sum  Inputs=+-  InputSameDT=on  SaturateOnIntegerOverflow=on  OutDataTypeStr=Inherit: Same as first input
  Stab : Outport  InitialOutput=0  VectorParamsAs1DForOutWhenUnconnected=off
  wires:
  Multiport Switch/1 -> Stab/1
  Generic Power System Stabilizer/1 -> Multiport Switch/3
  Sum2/1 -> Generic Power System Stabilizer/1
  Pm/1 -> Sum2/1
  Pe/1 -> Sum2/2
  Ground1/1 -> Multiport Switch/2
  [PSS_select] -> Multiport Switch/1
  dw/1 -> Multi-Band Power System Stabilizer/1
  Multi-Band Power System Stabilizer/1 -> Multiport Switch/4

== system GFM_29bus/North-West Network/Regulators4/Turbine  & Excitation Regulators Mac2/Stabilisateur ==
  Pm : Inport
  Pe : Inport  Port=2
  dw : Inport  Port=3
  Generic Power System Stabilizer : spsGenericPowerSystemStabilizerLib/Generic Power System Stabilizer  Tsensor=15e-3  K=2.5  Twashout=1  Tleadlag1="[0.06  1]"  Tleadlag2="[0  0]"  VSlimits=[-0.15 0.15]  Vinit=0  Plot_On=off  MagdB_On=on  FreqRange=logspace(-2,2,500)
      settings: SourceProductBaseCode=PS
  Ground1 : Ground
  Multi-Band Power System Stabilizer : spsMultiBandPowerSystemStabilizerLib/Multi-Band Power System Stabilizer  OperationMode=Simplified settings  Kg=0.7  GL=[0.2 10]  GI=[0.9 30]  GH=[12.0 115]  GLd=[66 66 9.4]  TcLF=[1.667 2 0 0 0 0 2 2.4 0 0 0 0 1 1]  GId=[66 66 47.6]  TcIF=[1 1 0.25 0.3 0 0 1 1 0.3 0.36 0 0 0 0]  GHd=[66 66 233]  TcHF="[0.01 0.012 0 0 0 0  0.012 0.0144 0 0 0 0 1 1]"  LIM=[.075 .15 .15 .15]  Plot_On=off  MagdB_On=on  FreqRange=logspace(-2,2,500)
      settings: SourceProductBaseCode=PS
  Multiport Switch : MultiPortSwitch  SaturateOnIntegerOverflow=on  InputSameDT=on
  Sum2 : Sum  Inputs=+-  InputSameDT=on  SaturateOnIntegerOverflow=on  OutDataTypeStr=Inherit: Same as first input
  Stab : Outport  InitialOutput=0  VectorParamsAs1DForOutWhenUnconnected=off
  wires:
  dw/1 -> Multi-Band Power System Stabilizer/1
  [PSS_select] -> Multiport Switch/1
  Ground1/1 -> Multiport Switch/2
  Pe/1 -> Sum2/2
  Pm/1 -> Sum2/1
  Sum2/1 -> Generic Power System Stabilizer/1
  Generic Power System Stabilizer/1 -> Multiport Switch/3
  Multiport Switch/1 -> Stab/1
  Multi-Band Power System Stabilizer/1 -> Multiport Switch/4
